simulink model "pendule_simple_perturbe"  (R2016a)
settings: Solver=VariableStepAuto  StartTime=0.0  StopTime=10  RelTol=1e-8
undefined symbols (not defined in the file): K, sigbuilder_block
libraries: simulink x1
settings Model: Creator=tmeunier  LastModifiedBy=tmeunier

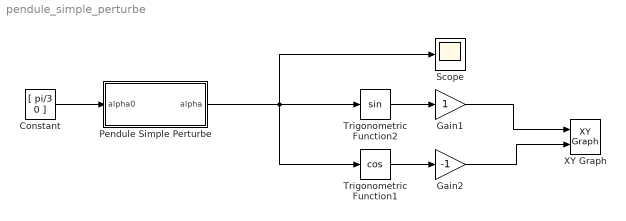
== system pendule_simple_perturbe ==
  Constant : Constant  Value=[ pi/3 0 ]
  Gain1 : Gain
  Gain2 : Gain  Gain=-1
  Pendule Simple Perturbe : Subsystem
  Scope : Scope
  Trigonometric Function1 : Trigonometry  Operator=cos
  Trigonometric Function2 : Trigonometry
  XY Graph : simulink/Sinks/XY Graph  xmin=-1  xmax=1  ymin=-1  ymax=1  st=-1
  wires:
  Gain1/1 -> XY Graph/1
  Trigonometric Function2/1 -> Gain1/1
  Trigonometric Function1/1 -> Gain2/1
  Gain2/1 -> XY Graph/2
  Pendule Simple Perturbe/1(alpha) -> Scope/1, Trigonometric Function1/1, Trigonometric Function2/1
  Constant/1 -> Pendule Simple Perturbe/1(alpha0)

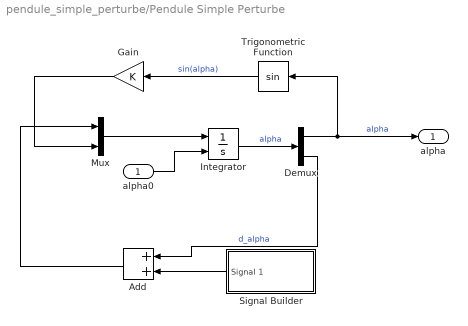
== system pendule_simple_perturbe/Pendule Simple Perturbe ==
  alpha0 : Inport
  Add : Sum
  Demux : Demux  Outputs=2
  Gain : Gain  Gain=K
  Integrator : Integrator  InitialConditionSource=external
  Mux : Mux  Inputs=2
  Signal Builder : Subsystem  Tag=STV Subsys  LoadFcn=sigbuilder_block('load');  StartFcn=sigbuilder_block('start');  StopFcn=sigbuilder_block('stop');  ClipboardFcn=sigbuilder_block('clipboard');  mask(Sigbuilder block){}
      mask help: Simulink:masks:SigbuilderBlock_MD
      mask init:
      | if ~strcmp(get_param(bdroot(gcbh),'SimulationStatus'),'stopped') tuvar = sigbuilder_block('maskInit'); end
      settings: CopyFcn=sigbuilder_block('copy');  DeleteFcn=sigbuilder_block('delete');  ModelCloseFcn=sigbuilder_block('modelClose');  PreSaveFcn=sigbuilder_block('preSave');  PauseFcn=sigbuilder_block('pause');  ContinueFcn=sigbuilder_block('continue');  NameChangeFcn=sigbuilder_block('namechange');  OpenFcn=sigbuilder_block('open',[437.305 199.326 550.989 400.168 ]);  CloseFcn=sigbuilder_block('close');
      mask Display: plot(0, 0, 100, 100,[2, 2, 32, 32, 2], [68, 8, 8, 68, 68],[32, 2], [38, 38], [32, 19, 2],[53, 60, 44], [32, 17, 17, 2],[16, 16, 31, 31]);txt = getActiveGroup(gcbh);text(2, 100, txt,'verticalAlignment', 'top');
  Trigonometric Function : Trigonometry
  alpha : Outport
  wires:
  Trigonometric Function/1 -> Gain/1  "sin(alpha)"
  alpha0/1 -> Integrator/2
  Integrator/1 -> Demux/1  "alpha"
  Demux/1 -> Trigonometric Function/1, alpha/1  "alpha"
  Gain/1 -> Mux/2
  Mux/1 -> Integrator/1
  Demux/2 -> Add/1  "d_alpha"
  Add/1 -> Mux/1
  Signal Builder/1(Signal 1) -> Add/2

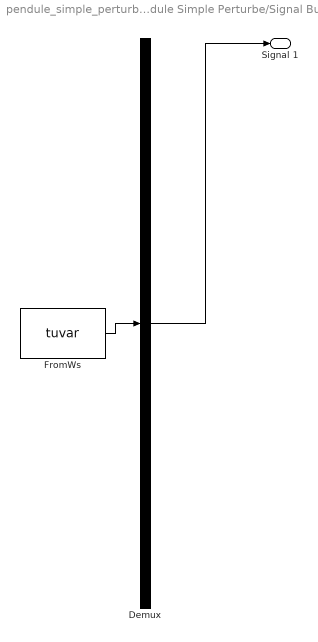
== system pendule_simple_perturbe/Pendule Simple Perturbe/Signal Builder ==
  Demux : Demux  Tag=STV Demux  Outputs=1
  FromWs : FromWorkspace  Tag=STV FromWs  VariableName=tuvar  SampleTime=0
      SigBuilderData=|
      | common.afterFinalStr = 'Extrapolate'
      | common.sampleTime = 0
      | dataSet.timeRange = [0 10]
      | dataSet.name = 'Group 1'
      | sbobj.Groups.Name = 'Group 1'
      | sbobj.Groups.Signals.Name = 'Signal 1'
      | sbobj.Groups.Signals.XData = [0 5 5 6 6 10]
      | sbobj.Groups.Signals.YData = [0 0 1 1 0 0]
  Signal 1 : Outport  Tag=STV Outport
  wires:
  Demux/1 -> Signal 1/1
  FromWs/1 -> Demux/1
